simulink model "sine_motor"  (Simulink 8.2)
settings: Solver=ode3  SolverMode=SingleTasking  StartTime=0.0  StopTime=15  FixedStep=ts1  RelTol=1e-3
InitFcn:
  | ts1 = 0.004;
  | a_d = 0.8;
  | Ts = 0.1;
libraries: legonxtlib x3
settings Model: Creator=Alphonso Monk  LastModifiedBy=Alphonso Monk  SimulationMode=external  ExtModeTrigDuration=2
settings DataIOCC: SignalLoggingSaveFormat=Dataset
settings OptimizationCC: ExpressionDepthLimit=128  OptimizeModelRefInitCode=on  LifeSpan=1
settings DebuggingCC: SolverPrmCheckMsg=none  FcnCallInpInsideContextMsg=EnableAllAsError  StateNameClashWarn=none
settings HardwareCC: ProdLargestAtomicInteger=Long  ProdLargestAtomicFloat=Float  ProdEndianess=LittleEndian  ProdHWDeviceType=ARM Compatible->ARM 7
settings RTWCC: SystemTargetFile=realtime.tlc  GenerateMakefile=off  TemplateMakefile=realtime.tmf  Description=Run on Target Hardware  RTWVerbose=off  ProcessScript=realtime_make_rtw_hook
settings STFCustomTargetCC: TargetLibSuffix=.a  CodeReplacementLibrary=ANSI_C  GenerateSampleERTMain=on  ERTCustomFileBanners=on  SupportNonInlinedSFcns=off  SupportVariableSizeSignals=on  MATLABClassNameForMDSCustomization=Simulink.SoftwareTarget.ERTCustomization  GRTInterface=off  SystemTargetFile=realtime.tlc
settings ERTTargetCC: CodeReplacementLibrary=ANSI_C  MultiwordLength=2048  GenerateSampleERTMain=on  ParMdlRefBuildCompliant=off  CompOptLevelCompliant=off  ConcurrentExecutionCompliant=off  CombineOutputUpdateFcns=off  ERTFirstTimeCompliant=off  SupportContinuousTime=on  SupportVariableSizeSignals=on  ModelStepFunctionPrototypeControlCompliant=off  CPPClassGenCompliant=off  ExtMode=on  ExtModeTransport=2  ExtModeMexArgs=0 5 9600 30  InlinedParameterPlacement=NonHierarchical  ERTSrcFileBannerTemplate=realtime_code_template.cgt  ERTHdrFileBannerTemplate=realtime_code_template.cgt  ERTDataSrcFileTemplate=realtime_code_template.cgt  ERTDataHdrFileTemplate=realtime_code_template.cgt  ERTCustomFileTemplate=realtime_file_process.tlc  ConvertIfToSwitch=off  SuppressUnreachableDefaultCases=off
settings SettingsController: Description=Run on Hardware Dialog  TargetExtensionPlatform=LEGO MINDSTORMS NXT
settings MATStruct: COM_port_number=1  Find_com_port=[0.0]  Enable_overrun_detection=[0.0]  Enable_LEGO_to_LEGO_communication=[0.0]  Bluetooth_mode=[1.0]  Slave_bluetooth_address=00:16:53:0f:0c:09

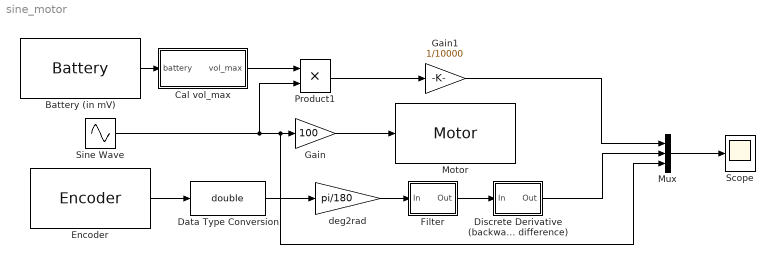
== system sine_motor ==
  Battery (in mV) : legonxtlib/Battery  sampleTime=Ts
  Cal vol_max : Subsystem
  Data Type Conversion : DataTypeConversion  OutDataTypeStr=double
  Discrete Derivative (backward difference) : Subsystem
  Encoder : legonxtlib/Encoder  portNumber=B  opMode=No reset  sampleTime=ts1
  Filter : Subsystem
  Gain : Gain  Gain=100
  Gain1 : Gain  Gain=1/10000
  Motor : legonxtlib/Motor  sportNumber=B  sstopAction=Brake
  Mux : Mux  Inputs=3
  Product1 : Product  Inputs=**
  Scope : Scope
      settings: SaveName=sineMotorResponse
  Sine Wave : Sin  Frequency=15  SampleTime=ts1
  deg2rad : Gain  Gain=pi/180  OutDataTypeStr=Inherit: Same as input  ParamDataTypeStr=Inherit: Same as input
  wires:
  Filter/1(Out) -> Discrete Derivative (backward difference)/1(In)
  deg2rad/1 -> Filter/1(In)
  Data Type Conversion/1 -> deg2rad/1
  Encoder/1 -> Data Type Conversion/1
  Mux/1 -> Scope/1
  Discrete Derivative (backward difference)/1(Out) -> Mux/2
  Sine Wave/1 -> Mux/3, Gain/1, Product1/2
  Cal vol_max/1(vol_max) -> Product1/1
  Battery (in mV)/1 -> Cal vol_max/1(battery)
  Gain/1 -> Motor/1
  Product1/1 -> Gain1/1
  Gain1/1 -> Mux/1

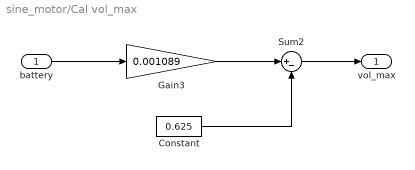
== system sine_motor/Cal vol_max ==
  battery : Inport
  Constant : Constant  Value=0.625  OutDataTypeStr=single
      settings: AttributesFormatString=DataType = %<OutDataTypeStr>
  Gain3 : Gain  Gain=0.001089  OutDataTypeStr=Inherit: Same as input  ParamDataTypeStr=Inherit: Same as input
  Sum2 : Sum  Inputs=|+-  OutDataTypeStr=Inherit: Same as first input
  vol_max : Outport
  wires:
  Gain3/1 -> Sum2/1
  Sum2/1 -> vol_max/1
  Constant/1 -> Sum2/2
  battery/1 -> Gain3/1

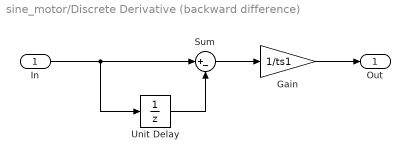
== system sine_motor/Discrete Derivative (backward difference) ==
  In : Inport
  Gain : Gain  Gain=1/ts1  OutDataTypeStr=Inherit: Same as input  ParamDataTypeStr=Inherit: Same as input
  Sum : Sum  Inputs=|+-  OutDataTypeStr=Inherit: Same as first input
  Unit Delay : UnitDelay  SampleTime=-1
  Out : Outport
  wires:
  Gain/1 -> Out/1
  In/1 -> Sum/1, Unit Delay/1
  Unit Delay/1 -> Sum/2
  Sum/1 -> Gain/1

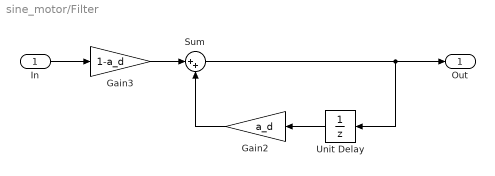
== system sine_motor/Filter ==
  In : Inport
  Gain2 : Gain  Gain=a_d  OutDataTypeStr=Inherit: Same as input  ParamDataTypeStr=Inherit: Same as input
  Gain3 : Gain  Gain=1-a_d  OutDataTypeStr=Inherit: Same as input  ParamDataTypeStr=Inherit: Same as input
  Sum : Sum  Inputs=|++  OutDataTypeStr=Inherit: Same as first input
  Unit Delay : UnitDelay  SampleTime=-1
  Out : Outport
  wires:
  In/1 -> Gain3/1
  Gain3/1 -> Sum/1
  Gain2/1 -> Sum/2
  Unit Delay/1 -> Gain2/1
  Sum/1 -> Out/1, Unit Delay/1
